simulink model "Hybrid_P2_Parallel"  (R2017b)
settings: Solver=FixedStepAuto  StartTime=0.0  StopTime=length(Speed)  FixedStep=0.01  MaxStep=0.01  RelTol=1e-3  EnableMultiTasking=on
PostLoadFcn:
  | , if any(exist('dsrtsu_mdlpostloadfcn', 'file') == [2, 3, 6]), try dsrtsu_mdlpostloadfcn('Execute', bdroot); catch fprintf('Error in PostLoadFcn (dsrtsu_mdlpostloadfcn) for model "%s":\n %s\n', bdroot, lasterr); end, end,
undefined symbols (not defined in the file): APP1_OOR, APP2_OOR, APP_Mismatch, Brk_Flt, cal, clt, Clutch, Clutch2, ClutchEngag, eng, Engine, EngOverTemp, ENGTRQ_MSMCH_Degraded_CP, ENGTRQ_MSMCH_ErrCritical_CP, ENGTRQ_MSMCH_LimpHome_CP, EngTrqMismatch, ess, ESSOverTemp, gb, KeyPos_Flt, LossCAN, MCUOverTemp, mot, MotDirMismatch, MotOverTemp, MotTrqMismatch, mph2kph, PRNDL_Flt, RegenFault, time, tloop
libraries: simulink x100, EC2_libraries x7, powerlib_meascontrol x2, lib_Actuators x1, CalculationGallon x1, lib_Chassis x1, autolibcoupling x1, autolibsharedcoupling x1, lib_DCDC x1, lib_Differential x1, lib_EMachine_2017a x1, lib_HVESS x1
(part 4 of 7)

== system Hybrid_P2_Parallel/Controller/HSC/Powertrain Manager/Torque Distribution/Supervisory  Control  Logic/VehReady.CS_Mode.Engine_Charge.Brake_mode1.MotTrqCalc1 ==
  note: Regenerative braking:
      | Regenerative braking should be allowed under specific chassis speed:
      | chas_spd_below_no_regen= 1.5;
      | chas_spd_above_full_regen = 3;
      | ess_soc_above_regen_forbidden = .92;  % ESS SOC above which regen braking is forbidden
      | ess_soc_above_regen_allowed = .9;% ESS SOC above which regen braking is allowed
  BPP : Inport
  VehSpd : Inport  Port=2
  ShftLvrPos : Inport  Port=3
  MotSpeed : Inport  Port=4
  TransRatio : Inport  Port=5
  IntdAxleTrq : Inport  Port=6
  f : TriggerPort  TriggerType=function-call  VariantControl=Variant
      settings: CopyFcn=Stateflow.SLINSF.SimulinkMan.removeBlockPreDeleteFcn  PreDeleteFcn=Stateflow.SLINSF.SimulinkMan.unsafePredeleteFcn
  "% to 1 " : Gain  Gain=1/100
  Constant : Constant  Value=0
  Constant1 : Constant  Value=0
  Constant2 : Constant  Value=fd.plant.init.ratio
  Divide : Product  Inputs=***
  Divide2 : Product  Inputs=***
  Index Vector : MultiPortSwitch  DataPortOrder=Zero-based contiguous  Inputs=5  zeroidx=on
  MinMax : MinMax  Function=max  Inputs=2
  Peak trq max - Regen : Lookup  InputValues=mot.plant.init.regen.trq_max.idx1_spd  Table=mot.plant.init.regen.trq_max.map  LookUpMeth=Interpolation-Use End Values  SaturateOnIntegerOverflow=on
  Regen Trq Derating1 : Lookup_n-D  NumberOfTableDimensions=1  BreakpointsForDimension1=[0 10 11 200]  Table=[0 0.5 1 1]  ExtrapMethod=Clip  UseLastTableValue=on  InternalRulePriority=Speed  RndMeth=Simplest  InputSameDT=on
  Regen_derat_overri : Constant  Value=0
  Regen_derat_value : Constant  Value=0.5
  Switch : Switch  Criteria=u2 > Threshold
  limit to 100Nm : Saturate  UpperLimit=0  LowerLimit=-100
  T : Outport
  wires:
  MinMax/1 -> [TrqCalc]
  IntdAxleTrq/1 -> MinMax/1
  Regen_derat_value/1 -> Switch/1
  Switch/1 -> Divide/3
  Regen_derat_overri/1 -> Switch/2
  Regen Trq Derating1/1 -> Switch/3
  Divide2/1 -> MinMax/2  "motor"
  TransRatio/1 -> Divide2/3
  limit to 100Nm/1 -> Divide2/2
  Constant2/1 -> Divide2/1
  Peak trq max - Regen/1 -> Divide/2
  MotSpeed/1 -> Peak trq max - Regen/1  "RPM"
  [TrqCalc] -> Index Vector/5  "N"
  Constant1/1 -> Index Vector/3  "P"
  Constant/1 -> Index Vector/2  "Between Ranges"
  Index Vector/1 -> T/1
  [TrqCalc] -> Index Vector/6  "D"
  [TrqCalc] -> Index Vector/4  "R"
  ShftLvrPos/1 -> Index Vector/1
  VehSpd/1 -> Regen Trq Derating1/1
  Divide/1 -> limit to 100Nm/1
  "% to 1 "/1 -> Divide/1
  BPP/1 -> "% to 1 "/1

== system Hybrid_P2_Parallel/Controller/HSC/Powertrain Manager/Torque Distribution/Supervisory  Control  Logic/VehReady.CS_Mode.Engine_Charge.Brake_mode1.MotTrqCalc2 ==
  note: Regenerative braking:
      | Regenerative braking should be allowed under specific chassis speed:
      | chas_spd_below_no_regen= 1.5;
      | chas_spd_above_full_regen = 3;
      | ess_soc_above_regen_forbidden = .92;  % ESS SOC above which regen braking is forbidden
      | ess_soc_above_regen_allowed = .9;% ESS SOC above which regen braking is allowed
  ShftLvrPos : Inport
  TransRatio : Inport  Port=2
  f : TriggerPort  TriggerType=function-call  VariantControl=Variant
      settings: CopyFcn=Stateflow.SLINSF.SimulinkMan.removeBlockPreDeleteFcn  PreDeleteFcn=Stateflow.SLINSF.SimulinkMan.unsafePredeleteFcn
  Constant : Constant  Value=0
  Constant1 : Constant  Value=0
  Constant2 : Constant  Value=fd.plant.init.ratio
  Divide2 : Product  Inputs=***
  Idle_torque_Regen : Constant  Value=0
  Index Vector : MultiPortSwitch  DataPortOrder=Zero-based contiguous  Inputs=5  zeroidx=on
  T : Outport
  wires:
  Idle_torque_Regen/1 -> Divide2/2
  Divide2/1 -> [TrqCalc]  "motor"
  TransRatio/1 -> Divide2/3
  Constant2/1 -> Divide2/1
  [TrqCalc] -> Index Vector/5  "N"
  Constant1/1 -> Index Vector/3  "P"
  Constant/1 -> Index Vector/2  "Between Ranges"
  Index Vector/1 -> T/1
  [TrqCalc] -> Index Vector/6  "D"
  [TrqCalc] -> Index Vector/4  "R"
  ShftLvrPos/1 -> Index Vector/1

== system Hybrid_P2_Parallel/Controller/HSC/Powertrain Manager/Torque Distribution/Supervisory  Control  Logic/VehReady.CS_Mode.Engine_Charge.Drive_Mode.EngTrq2EngApp ==
  Trq : Inport
  TransRatio : Inport  Port=2
  f : TriggerPort  TriggerType=function-call  VariantControl=Variant
      settings: CopyFcn=Stateflow.SLINSF.SimulinkMan.removeBlockPreDeleteFcn  PreDeleteFcn=Stateflow.SLINSF.SimulinkMan.unsafePredeleteFcn
  0-100% : Saturate  UpperLimit=100  LowerLimit=0
  Compare To Constant : simulink/Logic and Bit Operations/Compare To Constant  relop===  const=0  OutDataTypeStr=boolean
  Constant1 : Constant  Value=eps
  Constant5 : Constant  Value=fd.plant.init.ratio
  Divide1 : Product  Inputs=*//
  EngTrq2EngAPP : Lookup_n-D  NumberOfTableDimensions=1  BreakpointsForDimension1=[0:1:230]  Table="[-0.950562242591810\t-0.861179388327002\t-0.757792747831397\t-0.640901927898975\t-0.511000095283862\t-0.368573976700328\t-0.214103858822793\t-0.0480635882858183\t0.129079428315885\t0.316864224427463\t0.514836273533913\t0.722547489160089\t0.939556224870697\t1.16542727427030\t1.39973187100331\t1.64204768875400\t1.89195884124648\t2.14905588224475\t2.41293580555262\t2.68320204501379\t2.95946447451180\t3.24133940797003\t3.52844959935174\t3.82042424266002\t4.11689897193784\t4.41751586126800\t4.72192342477317\t5.02977661661586\t5.34073683099846\t5.65447190216317\t5.97065610439209\t6.28897015200715\t6.60910119937013\t6.93074284088268\t7.25359511098630\t7.57736448416234\t7.90176387493200\t8.22651263785634\t8.55133656753627\t8.87596789861257\t9.20014530576584\t9.52361390371657\t9.84612524722509\t10.1674373310916\t10.4873145901561\t10.8055278992985\t11.1218545734385\t11.4360783675358\t11.7479894765898\t12.0573845356398\t12.3640666197649\t12.6678452440843\t12.9685363637566\t13.2659623739808\t13.5599521099953\t13.8503408470787\t14.1369703005491\t14.4196886257647\t14.6983504181235\t14.9728167130634\t15.2429549860620\t15.5086391526369\t15.7697495683456\t16.0261730287853\t16.2778027695931\t16.5245384664460\t16.7662862350608\t17.0029586311942\t17.2344746506427\t17.4607597292427\t17.6817457428705\t17.8973710074422\t18.1075802789137\t18.3123247532808\t18.5115620665792\t18.7052562948843\t18.8933779543117\t19.0759040010164\t19.2528178311935\t19.4241092810781\t19.5897746269448\t19.7498165851084\t19.9042443119232\t20.0530734037837\t20.1963258971241\t20.3340302684184\t20.4662214341804\t20.5929407509641\t20.7142360153630\t20.8301614640105\t20.9407777735800\t21.0461520607847\t21.1463578823776\t21.2414752351516\t21.3315905559394\t21.4167967216136\t21.4971930490867\t21.5728852953111\t21.6439856572787\t21.7106127720217\t21.7728917166119\t21.8309540081611\t21.8849376038208\t21.9349869007824\t21.9812527362772\t22.0238923875764\t22.0630695719909\t22.0989544468717\t22.1317236096093\t22.1615600976344\t22.1886533884173\t22.2131993994684\t22.2354004883376\t22.2554654526151\t22.2736095299306\t22.2900543979538\t22.3050281743942\t22.3187654170013\t22.3315071235641\t22.3435007319120\t22.3550001199137\t22.3662656054781\t22.3775639465539\t22.3891683411296\t22.4013584272335\t22.4144202829338\t22.4286464263386\t22.4443358155959\t22.4617938488934\t22.4813323644587\t22.5032696405595\t22.5279303955028\t22.5556457876361\t22.5867534153463\t22.6215973170604\t22.6605279712450\t22.7039022964069\t22.7520836510924\t22.8054418338880\t22.8643530834197\t22.9292000783536\t23.0003719373956\t23.0782642192915\t23.1632789228268\t23.2558244868269\t23.3563157901571\t23.4651741517227\t23.5828273304686\t23.7097095253797\t23.8462613754808\t23.9929299598362\t24.1501687975506\t24.3184378477682\t24.4982035096730\t24.6899386224892\t24.8941224654804\t25.1112407579505\t25.3417856592430\t25.5862557687413\t25.8451561258686\t26.1189982100880\t26.4082999409026\t26.7135856778550\t27.0353862205281\t27.3742388085443\t27.7306871215661\t28.1052812792955\t28.4985778414748\t28.9111398078859\t29.3435366183506\t29.7963441527305\t30.2701447309271\t30.7655271128819\t31.2830864985759\t31.8234245280303\t32.3871492813060\t32.9748752785038\t33.5872234797643\t34.2248212852680\t34.8883025352352\t35.5783075099261\t36.2954829296408\t37.0404819547192\t37.8139641855409\t38.6165956625258\t39.4490488661331\t40.3120027168621\t41.2061425752523\t42.1321602418824\t43.0907539573713\t44.0826284023780\t45.1084946976008\t46.1690704037782\t47.2650795216887\t48.3972524921501\t49.5663261960208\t50.7730439541983\t52.0181555276205\t53.3024171172650\t54.6265913641491\t55.9914473493301\t57.3977605939052\t58.8463130590113\t60.3378931458253\t61.8732956955639\t63.4533219894835\t65.0787797488808\t66.7504831350916\t68.4692527494924\t70.2359156334991\t72.0513052685674\t73.9162615761929\t75.8316309179113\t77.7982660952979\t79.8170263499681\t81.8887773635766\t84.0143912578187\t86.1947465944290\t88.4307283751822\t90.7232280418928\t93.0731434764153\t95.4813790006436\t97.9488453765121\t100\t100\t100\t100\t100\t100\t100\t100]"  ExtrapMethod=Clip  UseLastTableValue=on  InternalRulePriority=Speed  RndMeth=Simplest  InputSameDT=on
  EngTrq2EngAPP_Linear : Lookup_n-D  NumberOfTableDimensions=1  BreakpointsForDimension1=[0:1:250]  Table=[0:0.4:100]  ExtrapMethod=Clip  UseLastTableValue=on  InternalRulePriority=Speed  RndMeth=Simplest  InputSameDT=on
  Switch : Switch  Criteria=u2 > Threshold
  APP : Outport
  wires:
  EngTrq2EngAPP_Linear/1 -> 0-100%/1  "EngTrq2EngAPP_CS"
  0-100%/1 -> APP/1
  TransRatio/1 -> Compare To Constant/1, Switch/3
  Divide1/1 -> EngTrq2EngAPP_Linear/1
  Switch/1 -> Divide1/3
  Constant1/1 -> Switch/1
  Compare To Constant/1 -> Switch/2
  Constant5/1 -> Divide1/2
  Trq/1 -> Divide1/1  "EngAxlTrqReq_CS"

== system Hybrid_P2_Parallel/Controller/HSC/Powertrain Manager/Torque Distribution/Supervisory  Control  Logic/VehReady.CS_Mode.Engine_Charge.Drive_Mode.EngTrqCalc ==
  EngSpeed : Inport
  APP : Inport  Port=2
  VehSpd : Inport  Port=3
  ShftLvrPos : Inport  Port=4
  DrvIntdAxleTrq : Inport  Port=5
  TransRatio : Inport  Port=6
  SOC : Inport  Port=7
  f : TriggerPort  TriggerType=function-call  VariantControl=Variant
      settings: CopyFcn=Stateflow.SLINSF.SimulinkMan.removeBlockPreDeleteFcn  PreDeleteFcn=Stateflow.SLINSF.SimulinkMan.unsafePredeleteFcn
  APP Derating : Lookup_n-D  NumberOfTableDimensions=1  BreakpointsForDimension1=[0 1 2 3 5 7]  Table=[0 0.1 0.3 0.5 0.7 1]  ExtrapMethod=Clip  UseLastTableValue=on  InternalRulePriority=Speed  RndMeth=Simplest  InputSameDT=on
  Constant : Constant  Value=0
  Constant1 : Constant  Value=0
  Constant3 : Constant  Value=fd.plant.init.ratio
  Divide : Product  Inputs=***
  Divide2 : Product  Inputs=***
  EngOptmTrq_Original : Lookup_n-D  NumberOfTableDimensions=1  BreakpointsForDimension1=[1550 1650 1850 2050 2350 2650 2950 3150 3250 3350]  Table="[154.020912669576\t173.623574282068\t180.662367834043\t186.327738253926\t182.858870786433\t180.175407273844\t178.037732950256\t181.891363533595\t190.985931710274\t199.537540592824]"  ExtrapMethod=Clip  UseLastTableValue=on  InternalRulePriority=Speed  RndMeth=Simplest  InputSameDT=on
  Engine Max Trq : Lookup_n-D  NumberOfTableDimensions=1  BreakpointsForDimension1="[600\t800\t1000\t1200\t1400\t1600\t1800\t2000\t2200\t2400\t2600\t2800\t3000\t3200\t3400\t3600\t3800\t4000\t4250\t4500\t4750\t5000\t5250\t5500\t5750\t6000\t6250\t6500]"  Table="[83.7900000000000\t136.760000000000\t140\t152.010000000000\t171.590000000000\t185.900000000000\t198.400000000000\t197.360000000000\t200.550000000000\t202.260000000000\t215.080000000000\t204.810000000000\t204.520000000000\t208.100000000000\t211.520000000000\t210.560000000000\t214.100000000000\t213.470000000000\t208.730000000000\t208.430000000000\t208.670000000000\t231.210000000000\t228.310000000000\t225.330000000000\t220.520000000000\t211.210000000000\t204.190000000000\t151.770000000000]"  ExtrapMethod=Clip  UseLastTableValue=on  InternalRulePriority=Speed  RndMeth=Simplest  InputSameDT=on
  MinMax : MinMax  Function=max  Inputs=2
  SOC Window Estimation : Subsystem
  Shifter : MultiPortSwitch  DataPortOrder=Zero-based contiguous  Inputs=5  zeroidx=on
  Switch : Switch  Criteria=u2 > Threshold
  VehSpd Derating : Lookup_n-D  NumberOfTableDimensions=1  BreakpointsForDimension1=[0 2 5]  Table=[0 0.5 1]  ExtrapMethod=Clip  UseLastTableValue=on  InternalRulePriority=Speed  RndMeth=Simplest  InputSameDT=on
  Trq : Outport
  EngActTRq : Outport  Port=2
  wires:
  MinMax/1 -> [TrqCalc]  "EngAxlTrqReq_CS"
  Constant3/1 -> Divide2/3
  TransRatio/1 -> Divide2/1
  EngOptmTrq_Original/1 -> Switch/3
  Engine Max Trq/1 -> Switch/1
  SOC Window Estimation/1(Out1) -> Switch/2
  SOC/1 -> SOC Window Estimation/1(SOC)
  Switch/1 -> Divide/1  "EngTrqAvl_CS"
  DrvIntdAxleTrq/1 -> MinMax/1  "DrvIntdAxlTrq_CS"
  Divide2/1 -> MinMax/2, EngActTRq/1  "EngAxlTrqAvl_CS"
  Divide/1 -> Divide2/2
  Shifter/1 -> Trq/1
  [TrqCalc] -> Shifter/5  "N"
  Constant1/1 -> Shifter/3  "P"
  Constant/1 -> Shifter/2  "Between Ranges"
  [TrqCalc] -> Shifter/6  "D"
  [TrqCalc] -> Shifter/4  "R"
  ShftLvrPos/1 -> Shifter/1
  VehSpd Derating/1 -> Divide/3  "VehSpeedDerating_CS"
  VehSpd/1 -> VehSpd Derating/1
  APP Derating/1 -> Divide/2  "APPDerating_CS"
  APP/1 -> APP Derating/1
  EngSpeed/1 -> Engine Max Trq/1, EngOptmTrq_Original/1

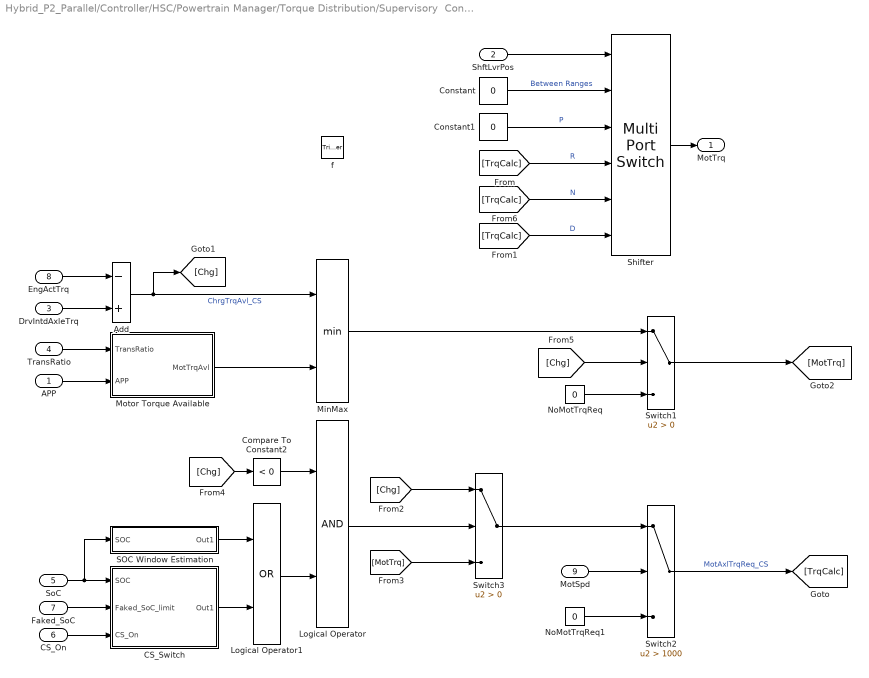
== system Hybrid_P2_Parallel/Controller/HSC/Powertrain Manager/Torque Distribution/Supervisory  Control  Logic/VehReady.CS_Mode.Engine_Charge.Drive_Mode.MotTrqCalc ==
  APP : Inport
  ShftLvrPos : Inport  Port=2
  DrvIntdAxleTrq : Inport  Port=3
  TransRatio : Inport  Port=4
  SoC : Inport  Port=5
  CS_On : Inport  Port=6
  Faked_SoC : Inport  Port=7
  EngActTrq : Inport  Port=8
  MotSpd : Inport  Port=9
  f : TriggerPort  TriggerType=function-call  VariantControl=Variant
      settings: CopyFcn=Stateflow.SLINSF.SimulinkMan.removeBlockPreDeleteFcn  PreDeleteFcn=Stateflow.SLINSF.SimulinkMan.unsafePredeleteFcn
  Add : Sum  Inputs=-+
  CS_Switch : Subsystem
  Compare To Constant2 : simulink/Logic and Bit Operations/Compare To Constant  relop=<  const=0  OutDataTypeStr=boolean
  Constant : Constant  Value=0
  Constant1 : Constant  Value=0
  Logical Operator : Logic  AllPortsSameDT=off  OutDataTypeStr=boolean
  Logical Operator1 : Logic  Operator=OR  AllPortsSameDT=off  OutDataTypeStr=boolean
  MinMax : MinMax  Inputs=2
  Motor Torque Available : Subsystem
  NoMotTrqReq : Constant  Value=0
  NoMotTrqReq1 : Constant  Value=0
  SOC Window Estimation : Subsystem
  Shifter : MultiPortSwitch  DataPortOrder=Zero-based contiguous  Inputs=5  zeroidx=on
  Switch1 : Switch  Criteria=u2 > Threshold
  Switch2 : Switch  Criteria=u2 > Threshold  Threshold=1000
  Switch3 : Switch  Criteria=u2 > Threshold
  MotTrq : Outport
  wires:
  [Chg] -> Switch1/2
  MotSpd/1 -> Switch2/2
  Motor Torque Available/1(MotTrqAvl) -> MinMax/2
  APP/1 -> Motor Torque Available/2(APP)
  TransRatio/1 -> Motor Torque Available/1(TransRatio)
  [Chg] -> Compare To Constant2/1
  [MotTrq] -> Switch3/3
  Switch1/1 -> [MotTrq]
  EngActTrq/1 -> Add/1
  Switch2/1 -> [TrqCalc]  "MotAxlTrqReq_CS"
  NoMotTrqReq1/1 -> Switch2/3
  CS_Switch/1(Out1) -> Logical Operator1/2
  CS_On/1 -> CS_Switch/3(CS_On)
  Faked_SoC/1 -> CS_Switch/2(Faked_SoC_limit)
  SOC Window Estimation/1(Out1) -> Logical Operator1/1
  Logical Operator1/1 -> Logical Operator/2
  Switch3/1 -> Switch2/1
  [Chg] -> Switch3/1
  Logical Operator/1 -> Switch3/2
  Compare To Constant2/1 -> Logical Operator/1
  NoMotTrqReq/1 -> Switch1/3
  MinMax/1 -> Switch1/1
  Add/1 -> MinMax/1, [Chg]  "ChrgTrqAvl_CS"
  SoC/1 -> CS_Switch/1(SOC), SOC Window Estimation/1(SOC)
  DrvIntdAxleTrq/1 -> Add/2
  Shifter/1 -> MotTrq/1
  [TrqCalc] -> Shifter/5  "N"
  Constant1/1 -> Shifter/3  "P"
  Constant/1 -> Shifter/2  "Between Ranges"
  [TrqCalc] -> Shifter/6  "D"
  [TrqCalc] -> Shifter/4  "R"
  ShftLvrPos/1 -> Shifter/1

== system Hybrid_P2_Parallel/Controller/HSC/Powertrain Manager/Torque Distribution/Supervisory  Control  Logic/VehReady.Clutch_Engage.SyncCtrl ==
  EngSpeed : Inport
  MotorSpeed : Inport  Port=2
  f : TriggerPort  TriggerType=function-call  VariantControl=Variant
      settings: CopyFcn=Stateflow.SLINSF.SimulinkMan.removeBlockPreDeleteFcn  PreDeleteFcn=Stateflow.SLINSF.SimulinkMan.unsafePredeleteFcn
  Kp : Gain  Gain=1/50
  Saturation1 : Saturate  UpperLimit=500  LowerLimit=-500
  Sum : Sum  Inputs=|+-
  EngApp : Outport
  wires:
  MotorSpeed/1 -> Sum/1  "RPM"
  EngSpeed/1 -> Sum/2
  Sum/1 -> Kp/1
  Kp/1 -> Saturation1/1
  Saturation1/1 -> EngApp/1

== system Hybrid_P2_Parallel/Controller/HSC/Powertrain Manager/Torque Distribution/Supervisory  Control  Logic/VehReady.Clutch_Engage1.SyncCtrl ==
  EngSpeed : Inport
  MotorSpeed : Inport  Port=2
  f : TriggerPort  TriggerType=function-call  VariantControl=Variant
      settings: CopyFcn=Stateflow.SLINSF.SimulinkMan.removeBlockPreDeleteFcn  PreDeleteFcn=Stateflow.SLINSF.SimulinkMan.unsafePredeleteFcn
  Kp : Gain  Gain=1/100
  Saturation : Saturate  UpperLimit=20  LowerLimit=0
  Sum : Sum  Inputs=|+-
  EngApp : Outport
  wires:
  MotorSpeed/1 -> Sum/1  "RPM"
  EngSpeed/1 -> Sum/2
  Sum/1 -> Kp/1
  Kp/1 -> Saturation/1
  Saturation/1 -> EngApp/1

== system Hybrid_P2_Parallel/Controller/HSC/Powertrain Manager/Torque Distribution/Supervisory  Control  Logic/VehReady.Clutch_Engage2.SyncCtrl ==
  EngSpeed : Inport
  MotorSpeed : Inport  Port=2
  f : TriggerPort  TriggerType=function-call  VariantControl=Variant
      settings: CopyFcn=Stateflow.SLINSF.SimulinkMan.removeBlockPreDeleteFcn  PreDeleteFcn=Stateflow.SLINSF.SimulinkMan.unsafePredeleteFcn
  Kp : Gain  Gain=1/100
  Saturation : Saturate  UpperLimit=20  LowerLimit=0
  Sum : Sum  Inputs=|+-
  EngApp : Outport
  wires:
  MotorSpeed/1 -> Sum/1  "RPM"
  EngSpeed/1 -> Sum/2
  Sum/1 -> Kp/1
  Kp/1 -> Saturation/1
  Saturation/1 -> EngApp/1

== system Hybrid_P2_Parallel/Controller/HSC/Powertrain Manager/Torque Distribution/Supervisory  Control  Logic/VehReady.Clutch_Engage3.SyncCtrl ==
  EngSpeed : Inport
  MotorSpeed : Inport  Port=2
  f : TriggerPort  TriggerType=function-call  VariantControl=Variant
      settings: CopyFcn=Stateflow.SLINSF.SimulinkMan.removeBlockPreDeleteFcn  PreDeleteFcn=Stateflow.SLINSF.SimulinkMan.unsafePredeleteFcn
  Kp : Gain  Gain=1/100
  Saturation : Saturate  UpperLimit=20  LowerLimit=0
  Sum : Sum  Inputs=|+-
  EngApp : Outport
  wires:
  MotorSpeed/1 -> Sum/1  "RPM"
  EngSpeed/1 -> Sum/2
  Sum/1 -> Kp/1
  Kp/1 -> Saturation/1
  Saturation/1 -> EngApp/1

== system Hybrid_P2_Parallel/Controller/HSC/Powertrain Manager/Torque Distribution/Supervisory  Control  Logic/VehReady.Eng_Charging_Stat.EngTrq2EngApp ==
  Trq : Inport
  TransRatio : Inport  Port=2
  f : TriggerPort  TriggerType=function-call  VariantControl=Variant
      settings: CopyFcn=Stateflow.SLINSF.SimulinkMan.removeBlockPreDeleteFcn  PreDeleteFcn=Stateflow.SLINSF.SimulinkMan.unsafePredeleteFcn
  Compare To Constant : simulink/Logic and Bit Operations/Compare To Constant  relop===  const=0  OutDataTypeStr=boolean
  Constant1 : Constant  Value=eps
  Constant5 : Constant  Value=fd.plant.init.ratio
  Divide1 : Product  Inputs=*//
  EngTrq2EngAPP : Lookup_n-D  NumberOfTableDimensions=1  BreakpointsForDimension1=[0:1:230]  Table="[-0.950562242591810\t-0.861179388327002\t-0.757792747831397\t-0.640901927898975\t-0.511000095283862\t-0.368573976700328\t-0.214103858822793\t-0.0480635882858183\t0.129079428315885\t0.316864224427463\t0.514836273533913\t0.722547489160089\t0.939556224870697\t1.16542727427030\t1.39973187100331\t1.64204768875400\t1.89195884124648\t2.14905588224475\t2.41293580555262\t2.68320204501379\t2.95946447451180\t3.24133940797003\t3.52844959935174\t3.82042424266002\t4.11689897193784\t4.41751586126800\t4.72192342477317\t5.02977661661586\t5.34073683099846\t5.65447190216317\t5.97065610439209\t6.28897015200715\t6.60910119937013\t6.93074284088268\t7.25359511098630\t7.57736448416234\t7.90176387493200\t8.22651263785634\t8.55133656753627\t8.87596789861257\t9.20014530576584\t9.52361390371657\t9.84612524722509\t10.1674373310916\t10.4873145901561\t10.8055278992985\t11.1218545734385\t11.4360783675358\t11.7479894765898\t12.0573845356398\t12.3640666197649\t12.6678452440843\t12.9685363637566\t13.2659623739808\t13.5599521099953\t13.8503408470787\t14.1369703005491\t14.4196886257647\t14.6983504181235\t14.9728167130634\t15.2429549860620\t15.5086391526369\t15.7697495683456\t16.0261730287853\t16.2778027695931\t16.5245384664460\t16.7662862350608\t17.0029586311942\t17.2344746506427\t17.4607597292427\t17.6817457428705\t17.8973710074422\t18.1075802789137\t18.3123247532808\t18.5115620665792\t18.7052562948843\t18.8933779543117\t19.0759040010164\t19.2528178311935\t19.4241092810781\t19.5897746269448\t19.7498165851084\t19.9042443119232\t20.0530734037837\t20.1963258971241\t20.3340302684184\t20.4662214341804\t20.5929407509641\t20.7142360153630\t20.8301614640105\t20.9407777735800\t21.0461520607847\t21.1463578823776\t21.2414752351516\t21.3315905559394\t21.4167967216136\t21.4971930490867\t21.5728852953111\t21.6439856572787\t21.7106127720217\t21.7728917166119\t21.8309540081611\t21.8849376038208\t21.9349869007824\t21.9812527362772\t22.0238923875764\t22.0630695719909\t22.0989544468717\t22.1317236096093\t22.1615600976344\t22.1886533884173\t22.2131993994684\t22.2354004883376\t22.2554654526151\t22.2736095299306\t22.2900543979538\t22.3050281743942\t22.3187654170013\t22.3315071235641\t22.3435007319120\t22.3550001199137\t22.3662656054781\t22.3775639465539\t22.3891683411296\t22.4013584272335\t22.4144202829338\t22.4286464263386\t22.4443358155959\t22.4617938488934\t22.4813323644587\t22.5032696405595\t22.5279303955028\t22.5556457876361\t22.5867534153463\t22.6215973170604\t22.6605279712450\t22.7039022964069\t22.7520836510924\t22.8054418338880\t22.8643530834197\t22.9292000783536\t23.0003719373956\t23.0782642192915\t23.1632789228268\t23.2558244868269\t23.3563157901571\t23.4651741517227\t23.5828273304686\t23.7097095253797\t23.8462613754808\t23.9929299598362\t24.1501687975506\t24.3184378477682\t24.4982035096730\t24.6899386224892\t24.8941224654804\t25.1112407579505\t25.3417856592430\t25.5862557687413\t25.8451561258686\t26.1189982100880\t26.4082999409026\t26.7135856778550\t27.0353862205281\t27.3742388085443\t27.7306871215661\t28.1052812792955\t28.4985778414748\t28.9111398078859\t29.3435366183506\t29.7963441527305\t30.2701447309271\t30.7655271128819\t31.2830864985759\t31.8234245280303\t32.3871492813060\t32.9748752785038\t33.5872234797643\t34.2248212852680\t34.8883025352352\t35.5783075099261\t36.2954829296408\t37.0404819547192\t37.8139641855409\t38.6165956625258\t39.4490488661331\t40.3120027168621\t41.2061425752523\t42.1321602418824\t43.0907539573713\t44.0826284023780\t45.1084946976008\t46.1690704037782\t47.2650795216887\t48.3972524921501\t49.5663261960208\t50.7730439541983\t52.0181555276205\t53.3024171172650\t54.6265913641491\t55.9914473493301\t57.3977605939052\t58.8463130590113\t60.3378931458253\t61.8732956955639\t63.4533219894835\t65.0787797488808\t66.7504831350916\t68.4692527494924\t70.2359156334991\t72.0513052685674\t73.9162615761929\t75.8316309179113\t77.7982660952979\t79.8170263499681\t81.8887773635766\t84.0143912578187\t86.1947465944290\t88.4307283751822\t90.7232280418928\t93.0731434764153\t95.4813790006436\t97.9488453765121\t100\t100\t100\t100\t100\t100\t100\t100]"  ExtrapMethod=Clip  UseLastTableValue=on  InternalRulePriority=Speed  RndMeth=Simplest  InputSameDT=on
  Saturation : Saturate  UpperLimit=100  LowerLimit=0
  Switch : Switch  Criteria=u2 > Threshold
  APP : Outport
  wires:
  Saturation/1 -> APP/1
  EngTrq2EngAPP/1 -> Saturation/1
  TransRatio/1 -> Compare To Constant/1, Switch/3
  Divide1/1 -> EngTrq2EngAPP/1
  Switch/1 -> Divide1/3
  Constant1/1 -> Switch/1
  Compare To Constant/1 -> Switch/2
  Constant5/1 -> Divide1/2
  Trq/1 -> Divide1/1

== system Hybrid_P2_Parallel/Controller/HSC/Powertrain Manager/Torque Distribution/Supervisory  Control  Logic/VehReady.Eng_Charging_Stat.EngTrqCalc ==
  EngSpeed : Inport
  ShftLvrPos : Inport  Port=2
  DrvIntdAxleTrq : Inport  Port=3
  TransRatio : Inport  Port=4
  f : TriggerPort  TriggerType=function-call  VariantControl=Variant
      settings: CopyFcn=Stateflow.SLINSF.SimulinkMan.removeBlockPreDeleteFcn  PreDeleteFcn=Stateflow.SLINSF.SimulinkMan.unsafePredeleteFcn
  Constant{,1..2,4} (4 alike) : Constant  Value=0
  Constant3 : Constant  Value=fd.plant.init.ratio
  Divide2 : Product  Inputs=***
  Engine Max Trq : Lookup_n-D  NumberOfTableDimensions=1  BreakpointsForDimension1="[600\t800\t1000\t1200\t1400\t1600\t1800\t2000\t2200\t2400\t2600\t2800\t3000\t3200\t3400\t3600\t3800\t4000\t4250\t4500\t4750\t5000\t5250\t5500\t5750\t6000\t6250\t6500]"  Table="[83.7900000000000\t136.760000000000\t140\t152.010000000000\t171.590000000000\t185.900000000000\t198.400000000000\t197.360000000000\t200.550000000000\t202.260000000000\t215.080000000000\t204.810000000000\t204.520000000000\t208.100000000000\t211.520000000000\t210.560000000000\t214.100000000000\t213.470000000000\t208.730000000000\t208.430000000000\t208.670000000000\t231.210000000000\t228.310000000000\t225.330000000000\t220.520000000000\t211.210000000000\t204.190000000000\t151.770000000000]"  ExtrapMethod=Clip  UseLastTableValue=on  InternalRulePriority=Speed  RndMeth=Simplest  InputSameDT=on
  MinMax : MinMax  Function=max  Inputs=2
  Multiply by Zero Fix : Subsystem
  Shifter : MultiPortSwitch  DataPortOrder=Zero-based contiguous  Inputs=5  zeroidx=on
  Trq : Outport
  wires:
  Multiply by Zero Fix/1(Out1) -> Divide2/3
  TransRatio/1 -> Multiply by Zero Fix/1(In1)
  MinMax/1 -> [TrqCalc]
  DrvIntdAxleTrq/1 -> MinMax/1  "driver"
  Divide2/1 -> MinMax/2  "engine"
  Engine Max Trq/1 -> Divide2/2
  Constant3/1 -> Divide2/1
  Shifter/1 -> Trq/1
  Constant2/1 -> Shifter/5  "N"
  [TrqCalc] -> Shifter/3  "P"
  Constant/1 -> Shifter/2  "Between Ranges"
  Constant4/1 -> Shifter/6  "D"
  Constant1/1 -> Shifter/4  "R"
  ShftLvrPos/1 -> Shifter/1
  EngSpeed/1 -> Engine Max Trq/1

== system Hybrid_P2_Parallel/Controller/HSC/Powertrain Manager/Torque Distribution/Supervisory  Control  Logic/VehReady.Eng_Charging_Stat.MotTrqCalc ==
  ShftLvrPos : Inport
  DrvIntdAxleTrq : Inport  Port=2
  Trq : Inport  Port=3
  f : TriggerPort  TriggerType=function-call  VariantControl=Variant
      settings: CopyFcn=Stateflow.SLINSF.SimulinkMan.removeBlockPreDeleteFcn  PreDeleteFcn=Stateflow.SLINSF.SimulinkMan.unsafePredeleteFcn
  Add : Sum  Inputs=-+
  Constant{,1..3} (4 alike) : Constant  Value=0
  Goto : Goto  Commented=on  GotoTag=TrqCalc
  NoMotTrqReq : Constant  Commented=on  Value=0
  Saturation : Saturate  UpperLimit=100  LowerLimit=-inf
  Shifter : MultiPortSwitch  DataPortOrder=Zero-based contiguous  Inputs=5  zeroidx=on
  Switch1 : Switch  Commented=on  Criteria=u2 > Threshold
  MotTrq : Outport
  wires:
  Saturation/1 -> [TrqCalc]
  Add/1 -> Switch1/2, Switch1/1, Saturation/1
  Switch1/1 -> Goto/1
  Trq/1 -> Add/1
  NoMotTrqReq/1 -> Switch1/3
  DrvIntdAxleTrq/1 -> Add/2
  Shifter/1 -> MotTrq/1
  Constant2/1 -> Shifter/5  "N"
  [TrqCalc] -> Shifter/3  "P"
  Constant/1 -> Shifter/2  "Between Ranges"
  Constant3/1 -> Shifter/6  "D"
  Constant1/1 -> Shifter/4  "R"
  ShftLvrPos/1 -> Shifter/1

== system Hybrid_P2_Parallel/Controller/HSC/Powertrain Manager/Torque Distribution/Supervisory  Control  Logic/VehReady.Eng_Only_Mode.EngTrq2EngApp ==
  T : Inport
  TransRatio : Inport  Port=2
  f : TriggerPort  TriggerType=function-call  VariantControl=Variant
      settings: CopyFcn=Stateflow.SLINSF.SimulinkMan.removeBlockPreDeleteFcn  PreDeleteFcn=Stateflow.SLINSF.SimulinkMan.unsafePredeleteFcn
  0-100% : Saturate  UpperLimit=100  LowerLimit=0
  Compare To Constant : simulink/Logic and Bit Operations/Compare To Constant  relop===  const=0  OutDataTypeStr=boolean
  Constant1 : Constant  Value=eps
  Constant5 : Constant  Value=fd.plant.init.ratio
  Divide by 0 Fix : Switch  Criteria=u2 > Threshold
  Divide1 : Product  Inputs=*//
  EngTrq2EngAPP : Lookup_n-D  NumberOfTableDimensions=1  BreakpointsForDimension1=[0:1:230]  Table="[-0.950562242591810\t-0.861179388327002\t-0.757792747831397\t-0.640901927898975\t-0.511000095283862\t-0.368573976700328\t-0.214103858822793\t-0.0480635882858183\t0.129079428315885\t0.316864224427463\t0.514836273533913\t0.722547489160089\t0.939556224870697\t1.16542727427030\t1.39973187100331\t1.64204768875400\t1.89195884124648\t2.14905588224475\t2.41293580555262\t2.68320204501379\t2.95946447451180\t3.24133940797003\t3.52844959935174\t3.82042424266002\t4.11689897193784\t4.41751586126800\t4.72192342477317\t5.02977661661586\t5.34073683099846\t5.65447190216317\t5.97065610439209\t6.28897015200715\t6.60910119937013\t6.93074284088268\t7.25359511098630\t7.57736448416234\t7.90176387493200\t8.22651263785634\t8.55133656753627\t8.87596789861257\t9.20014530576584\t9.52361390371657\t9.84612524722509\t10.1674373310916\t10.4873145901561\t10.8055278992985\t11.1218545734385\t11.4360783675358\t11.7479894765898\t12.0573845356398\t12.3640666197649\t12.6678452440843\t12.9685363637566\t13.2659623739808\t13.5599521099953\t13.8503408470787\t14.1369703005491\t14.4196886257647\t14.6983504181235\t14.9728167130634\t15.2429549860620\t15.5086391526369\t15.7697495683456\t16.0261730287853\t16.2778027695931\t16.5245384664460\t16.7662862350608\t17.0029586311942\t17.2344746506427\t17.4607597292427\t17.6817457428705\t17.8973710074422\t18.1075802789137\t18.3123247532808\t18.5115620665792\t18.7052562948843\t18.8933779543117\t19.0759040010164\t19.2528178311935\t19.4241092810781\t19.5897746269448\t19.7498165851084\t19.9042443119232\t20.0530734037837\t20.1963258971241\t20.3340302684184\t20.4662214341804\t20.5929407509641\t20.7142360153630\t20.8301614640105\t20.9407777735800\t21.0461520607847\t21.1463578823776\t21.2414752351516\t21.3315905559394\t21.4167967216136\t21.4971930490867\t21.5728852953111\t21.6439856572787\t21.7106127720217\t21.7728917166119\t21.8309540081611\t21.8849376038208\t21.9349869007824\t21.9812527362772\t22.0238923875764\t22.0630695719909\t22.0989544468717\t22.1317236096093\t22.1615600976344\t22.1886533884173\t22.2131993994684\t22.2354004883376\t22.2554654526151\t22.2736095299306\t22.2900543979538\t22.3050281743942\t22.3187654170013\t22.3315071235641\t22.3435007319120\t22.3550001199137\t22.3662656054781\t22.3775639465539\t22.3891683411296\t22.4013584272335\t22.4144202829338\t22.4286464263386\t22.4443358155959\t22.4617938488934\t22.4813323644587\t22.5032696405595\t22.5279303955028\t22.5556457876361\t22.5867534153463\t22.6215973170604\t22.6605279712450\t22.7039022964069\t22.7520836510924\t22.8054418338880\t22.8643530834197\t22.9292000783536\t23.0003719373956\t23.0782642192915\t23.1632789228268\t23.2558244868269\t23.3563157901571\t23.4651741517227\t23.5828273304686\t23.7097095253797\t23.8462613754808\t23.9929299598362\t24.1501687975506\t24.3184378477682\t24.4982035096730\t24.6899386224892\t24.8941224654804\t25.1112407579505\t25.3417856592430\t25.5862557687413\t25.8451561258686\t26.1189982100880\t26.4082999409026\t26.7135856778550\t27.0353862205281\t27.3742388085443\t27.7306871215661\t28.1052812792955\t28.4985778414748\t28.9111398078859\t29.3435366183506\t29.7963441527305\t30.2701447309271\t30.7655271128819\t31.2830864985759\t31.8234245280303\t32.3871492813060\t32.9748752785038\t33.5872234797643\t34.2248212852680\t34.8883025352352\t35.5783075099261\t36.2954829296408\t37.0404819547192\t37.8139641855409\t38.6165956625258\t39.4490488661331\t40.3120027168621\t41.2061425752523\t42.1321602418824\t43.0907539573713\t44.0826284023780\t45.1084946976008\t46.1690704037782\t47.2650795216887\t48.3972524921501\t49.5663261960208\t50.7730439541983\t52.0181555276205\t53.3024171172650\t54.6265913641491\t55.9914473493301\t57.3977605939052\t58.8463130590113\t60.3378931458253\t61.8732956955639\t63.4533219894835\t65.0787797488808\t66.7504831350916\t68.4692527494924\t70.2359156334991\t72.0513052685674\t73.9162615761929\t75.8316309179113\t77.7982660952979\t79.8170263499681\t81.8887773635766\t84.0143912578187\t86.1947465944290\t88.4307283751822\t90.7232280418928\t93.0731434764153\t95.4813790006436\t97.9488453765121\t100\t100\t100\t100\t100\t100\t100\t100]"  ExtrapMethod=Clip  UseLastTableValue=on  InternalRulePriority=Speed  RndMeth=Simplest  InputSameDT=on
  APP : Outport
  wires:
  0-100%/1 -> APP/1
  EngTrq2EngAPP/1 -> 0-100%/1
  TransRatio/1 -> Compare To Constant/1, Divide by 0 Fix/3
  Divide1/1 -> EngTrq2EngAPP/1
  Divide by 0 Fix/1 -> Divide1/3
  Constant1/1 -> Divide by 0 Fix/1
  Compare To Constant/1 -> Divide by 0 Fix/2
  Constant5/1 -> Divide1/2
  T/1 -> Divide1/1

== system Hybrid_P2_Parallel/Controller/HSC/Powertrain Manager/Torque Distribution/Supervisory  Control  Logic/VehReady.Eng_Only_Mode.EngTrqCalc ==
  APP : Inport
  EngSpeed : Inport  Port=2
  Shifter : Inport  Port=3
  DrvIntdAxleTrq : Inport  Port=4
  TransRatio : Inport  Port=5
  f : TriggerPort  TriggerType=function-call  VariantControl=Variant
      settings: CopyFcn=Stateflow.SLINSF.SimulinkMan.removeBlockPreDeleteFcn  PreDeleteFcn=Stateflow.SLINSF.SimulinkMan.unsafePredeleteFcn
  Constant : Constant  Value=0
  Constant1 : Constant  Value=0
  Constant2 : Constant  Value=0
  Divide2 : Product  Inputs=**
  Divide3 : Product  Inputs=***
  Engine Max Trq : Lookup_n-D  NumberOfTableDimensions=1  BreakpointsForDimension1="[600\t800\t1000\t1200\t1400\t1600\t1800\t2000\t2200\t2400\t2600\t2800\t3000\t3200\t3400\t3600\t3800\t4000\t4250\t4500\t4750\t5000\t5250\t5500\t5750\t6000\t6250\t6500]"  Table="[83.7900000000000\t136.760000000000\t140\t152.010000000000\t171.590000000000\t185.900000000000\t198.400000000000\t197.360000000000\t200.550000000000\t202.260000000000\t215.080000000000\t204.810000000000\t204.520000000000\t208.100000000000\t211.520000000000\t210.560000000000\t214.100000000000\t213.470000000000\t208.730000000000\t208.430000000000\t208.670000000000\t231.210000000000\t228.310000000000\t225.330000000000\t220.520000000000\t211.210000000000\t204.190000000000\t151.770000000000]"  ExtrapMethod=Clip  UseLastTableValue=on  InternalRulePriority=Speed  RndMeth=Simplest  InputSameDT=on
  Final Drive Ratio1 : Constant  Value=fd.plant.init.ratio
  Gain : Gain  Gain=1/100
  Index Vector : MultiPortSwitch  DataPortOrder=Zero-based contiguous  Inputs=5  zeroidx=on
  MinMax : MinMax  Inputs=2
  T : Outport
  wires:
  MinMax/1 -> [TrqCalc]
  DrvIntdAxleTrq/1 -> MinMax/2
  Divide3/1 -> MinMax/1
  Final Drive Ratio1/1 -> Divide3/3
  TransRatio/1 -> Divide3/2
  Divide2/1 -> Divide3/1
  Engine Max Trq/1 -> Divide2/2
  EngSpeed/1 -> Engine Max Trq/1  "RPM"
  Gain/1 -> Divide2/1
  APP/1 -> Gain/1
  Shifter/1 -> Index Vector/1
  Index Vector/1 -> T/1
  Constant2/1 -> Index Vector/5  "N"
  Constant1/1 -> Index Vector/3  "P"
  Constant/1 -> Index Vector/2  "Between Ranges"
  [TrqCalc] -> Index Vector/6  "D"
  [TrqCalc] -> Index Vector/4  "R"

== system Hybrid_P2_Parallel/Controller/HSC/Powertrain Manager/Torque Distribution/Supervisory  Control  Logic/VehReady.Sport_Mode.Brake_mode.MotTrqCalc1 ==
  note: Regenerative braking:
      | Regenerative braking should be allowed under specific chassis speed:
      | chas_spd_below_no_regen= 1.5;
      | chas_spd_above_full_regen = 3;
      | ess_soc_above_regen_forbidden = .92;  % ESS SOC above which regen braking is forbidden
      | ess_soc_above_regen_allowed = .9;% ESS SOC above which regen braking is allowed
  BPP : Inport
  VehSpd : Inport  Port=2
  ShftLvrPos : Inport  Port=3
  MotSpeed : Inport  Port=4
  IntdAxleTrq : Inport  Port=5
  TransRatio : Inport  Port=6
  f : TriggerPort  TriggerType=function-call  VariantControl=Variant
      settings: CopyFcn=Stateflow.SLINSF.SimulinkMan.removeBlockPreDeleteFcn  PreDeleteFcn=Stateflow.SLINSF.SimulinkMan.unsafePredeleteFcn
  "% to 1 " : Gain  Gain=1/100
  Constant : Constant  Value=0
  Constant1 : Constant  Value=0
  Constant2 : Constant  Value=fd.plant.init.ratio
  Divide : Product  Inputs=***
  Divide2 : Product  Inputs=***
  Index Vector : MultiPortSwitch  DataPortOrder=Zero-based contiguous  Inputs=5  zeroidx=on
  MinMax : MinMax  Function=max  Inputs=2
  Peak trq max - Regen : Lookup  InputValues=mot.plant.init.regen.trq_max.idx1_spd  Table=mot.plant.init.regen.trq_max.map  LookUpMeth=Interpolation-Use End Values  SaturateOnIntegerOverflow=on
  Regen Trq Derating : Lookup_n-D  NumberOfTableDimensions=1  BreakpointsForDimension1=[0 10 20 30 40]  Table=[0 0.025 0.05 0.1 1]  ExtrapMethod=Clip  UseLastTableValue=on  InternalRulePriority=Speed  RndMeth=Simplest  InputSameDT=on
  limit to 200Nm : Saturate  UpperLimit=0  LowerLimit=-200
  T : Outport
  wires:
  Regen Trq Derating/1 -> Divide/3
  MinMax/1 -> [TrqCalc]
  Divide2/1 -> MinMax/2  "motor"
  IntdAxleTrq/1 -> MinMax/1
  TransRatio/1 -> Divide2/3
  limit to 200Nm/1 -> Divide2/2
  Constant2/1 -> Divide2/1
  Peak trq max - Regen/1 -> Divide/2
  MotSpeed/1 -> Peak trq max - Regen/1  "RPM"
  [TrqCalc] -> Index Vector/5  "N"
  Constant1/1 -> Index Vector/3  "P"
  Constant/1 -> Index Vector/2  "Between Ranges"
  Index Vector/1 -> T/1
  [TrqCalc] -> Index Vector/6  "D"
  [TrqCalc] -> Index Vector/4  "R"
  ShftLvrPos/1 -> Index Vector/1
  VehSpd/1 -> Regen Trq Derating/1
  Divide/1 -> limit to 200Nm/1
  "% to 1 "/1 -> Divide/1
  BPP/1 -> "% to 1 "/1

== system Hybrid_P2_Parallel/Controller/HSC/Powertrain Manager/Torque Distribution/Supervisory  Control  Logic/VehReady.Sport_Mode.EngTrq2EngApp ==
  note: Change pedal map
  Trq : Inport
  TransRatio : Inport  Port=2
  f : TriggerPort  TriggerType=function-call  VariantControl=Variant
      settings: CopyFcn=Stateflow.SLINSF.SimulinkMan.removeBlockPreDeleteFcn  PreDeleteFcn=Stateflow.SLINSF.SimulinkMan.unsafePredeleteFcn
  0-100% : Saturate  UpperLimit=100  LowerLimit=0
  Compare To Constant : simulink/Logic and Bit Operations/Compare To Constant  relop===  const=0  OutDataTypeStr=boolean
  Constant1 : Constant  Value=eps
  Constant5 : Constant  Value=fd.plant.init.ratio
  Divide by 0 Fix : Switch  Criteria=u2 > Threshold
  Divide1 : Product  Inputs=*//
  EngTrq2EngAPP_Linear : Lookup_n-D  NumberOfTableDimensions=1  BreakpointsForDimension1=[0:1:200]  Table=[0:0.5:100]  ExtrapMethod=Clip  UseLastTableValue=on  InternalRulePriority=Speed  RndMeth=Simplest  InputSameDT=on
  APP : Outport
  wires:
  EngTrq2EngAPP_Linear/1 -> 0-100%/1
  0-100%/1 -> APP/1
  TransRatio/1 -> Compare To Constant/1, Divide by 0 Fix/3
  Divide1/1 -> EngTrq2EngAPP_Linear/1
  Divide by 0 Fix/1 -> Divide1/3
  Constant1/1 -> Divide by 0 Fix/1
  Compare To Constant/1 -> Divide by 0 Fix/2
  Constant5/1 -> Divide1/2
  Trq/1 -> Divide1/1

== system Hybrid_P2_Parallel/Controller/HSC/Powertrain Manager/Torque Distribution/Supervisory  Control  Logic/VehReady.Sport_Mode.EngTrqCalc ==
  APP : Inport
  EngSpeed : Inport  Port=2
  Shifter : Inport  Port=3
  DrvIntdAxleTrq : Inport  Port=4
  TransRatio : Inport  Port=5
  f : TriggerPort  TriggerType=function-call  VariantControl=Variant
      settings: CopyFcn=Stateflow.SLINSF.SimulinkMan.removeBlockPreDeleteFcn  PreDeleteFcn=Stateflow.SLINSF.SimulinkMan.unsafePredeleteFcn
  Constant : Constant  Value=0
  Constant1 : Constant  Value=0
  Divide2 : Product  Inputs=**
  Divide3 : Product  Inputs=***
  Engine Max Trq : Lookup_n-D  NumberOfTableDimensions=1  BreakpointsForDimension1="[600\t800\t1000\t1200\t1400\t1600\t1800\t2000\t2200\t2400\t2600\t2800\t3000\t3200\t3400\t3600\t3800\t4000\t4250\t4500\t4750\t5000\t5250\t5500\t5750\t6000\t6250\t6500]"  Table="[83.7900000000000\t136.760000000000\t140\t152.010000000000\t171.590000000000\t185.900000000000\t198.400000000000\t197.360000000000\t200.550000000000\t202.260000000000\t215.080000000000\t204.810000000000\t204.520000000000\t208.100000000000\t211.520000000000\t210.560000000000\t214.100000000000\t213.470000000000\t208.730000000000\t208.430000000000\t208.670000000000\t231.210000000000\t228.310000000000\t225.330000000000\t220.520000000000\t211.210000000000\t204.190000000000\t151.770000000000]"  ExtrapMethod=Clip  UseLastTableValue=on  InternalRulePriority=Speed  RndMeth=Simplest  InputSameDT=on
  Final Drive Ratio : Constant  Value=fd.plant.init.ratio
  Index Vector : MultiPortSwitch  DataPortOrder=Zero-based contiguous  Inputs=5  zeroidx=on
  MinMax : MinMax  Inputs=2
  Saturation : Saturate  UpperLimit=230  LowerLimit=-inf
  to% : Gain  Gain=1/100
  T : Outport
  wires:
  [TrqCalc] -> Index Vector/4  "R"
  [TrqCalc] -> Index Vector/6  "D"
  Constant/1 -> Index Vector/2  "Between Ranges"
  Constant1/1 -> Index Vector/3  "P"
  [TrqCalc] -> Index Vector/5  "N"
  Index Vector/1 -> T/1
  Shifter/1 -> Index Vector/1
  APP/1 -> to%/1
  to%/1 -> Divide2/1
  EngSpeed/1 -> Engine Max Trq/1  "RPM"
  Engine Max Trq/1 -> Saturation/1
  Saturation/1 -> Divide2/2
  Divide2/1 -> Divide3/1
  TransRatio/1 -> Divide3/2
  Final Drive Ratio/1 -> Divide3/3
  Divide3/1 -> MinMax/1
  DrvIntdAxleTrq/1 -> MinMax/2
  MinMax/1 -> [TrqCalc]

== system Hybrid_P2_Parallel/Controller/HSC/Powertrain Manager/Torque Distribution/Supervisory  Control  Logic/VehReady.Sport_Mode.MotTrqCalc ==
  APP : Inport
  Shifter : Inport  Port=2
  MotSpeed : Inport  Port=3
  DrvIntdAxleTrq : Inport  Port=4
  TransRatio : Inport  Port=5
  f : TriggerPort  TriggerType=function-call  VariantControl=Variant
      settings: CopyFcn=Stateflow.SLINSF.SimulinkMan.removeBlockPreDeleteFcn  PreDeleteFcn=Stateflow.SLINSF.SimulinkMan.unsafePredeleteFcn
  % to 1 : Gain  Gain=1/100
  Constant : Constant  Value=0
  Constant1 : Constant  Value=0
  Differential Ratio : Constant  Value=fd.plant.init.ratio
  Divide1 : Product  Inputs=**
  Divide2 : Product  Inputs=***
  Index Vector : MultiPortSwitch  DataPortOrder=Zero-based contiguous  Inputs=5  zeroidx=on
  MinMax : MinMax  Inputs=2
  Peak trq max - Motoring : Lookup  InputValues=mot.plant.init.regen.trq_max.idx1_spd  Table=mot.plant.init.motor.trq_max.map  LookUpMeth=Interpolation-Use End Values  SaturateOnIntegerOverflow=on
  T : Outport
  wires:
  % to 1/1 -> Divide1/2
  Shifter/1 -> Index Vector/1
  [TrqCalc] -> Index Vector/4  "R"
  [TrqCalc] -> Index Vector/6  "D"
  Index Vector/1 -> T/1
  Constant/1 -> Index Vector/2  "Between Ranges"
  Constant1/1 -> Index Vector/3  "P"
  [TrqCalc] -> Index Vector/5  "N"
  APP/1 -> % to 1/1
  MotSpeed/1 -> Peak trq max - Motoring/1  "RPM"
  Peak trq max - Motoring/1 -> Divide1/1
  Divide1/1 -> Divide2/1
  TransRatio/1 -> Divide2/2
  Differential Ratio/1 -> Divide2/3
  DrvIntdAxleTrq/1 -> MinMax/1
  Divide2/1 -> MinMax/2
  MinMax/1 -> [TrqCalc]

== system Hybrid_P2_Parallel/Controller/HSC/Powertrain Manager/Torque Distribution/SysPwrMd ==
  note: Switch added to test engine start
      | 04/13/2017 - Sebastian
  note: Disable Engine if HVIL on
  SysPwrMd : Inport
  EngRunAtv : Inport  Port=2
  EngOnReq : Inport  Port=3
  Fehler_Pilot : Inport  Port=4
  Constant1 : Constant  Value=3
  Constant2 : Constant
  Constant3 : Constant  Value=0
  EngOnReq_Cal : Constant  Value=0
  Saturation2 : Saturate  UpperLimit=2  LowerLimit=0
  Saturation3 : Saturate  UpperLimit=2  LowerLimit=0
  Switch{1..5} (5 alike) : Switch  Threshold=1
  Out1 : Outport
  wires:
  Constant3/1 -> Switch5/1
  Switch5/1 -> Out1/1
  Fehler_Pilot/1 -> Switch5/2
  Switch4/1 -> Switch3/2
  EngOnReq_Cal/1 -> Switch4/1, Switch4/2
  Switch3/1 -> Switch5/3
  Switch1/1 -> Switch3/1
  EngOnReq/1 -> Switch4/3
  Saturation3/1 -> Switch2/3
  SysPwrMd/1 -> Saturation2/1, Saturation3/1
  Saturation2/1 -> Switch1/1
  EngRunAtv/1 -> Switch1/2, Switch2/2
  Constant2/1 -> Switch2/1
  Constant1/1 -> Switch1/3
  Switch2/1 -> Switch3/3

== system Hybrid_P2_Parallel/Controller/HSC/Powertrain Manager/Torque Distribution/eSystemStatusValidity ==
  In1 : Inport
  " Normal Operation" : simulink/Logic and Bit Operations/Compare To Constant  relop===  const=2  OutDataTypeStr=boolean
  Limited Operation : simulink/Logic and Bit Operations/Compare To Constant  relop===  const=1  OutDataTypeStr=boolean
  Logical Operator : Logic  Operator=OR  AllPortsSameDT=off  OutDataTypeStr=boolean
  Out1 : Outport
  wires:
  Logical Operator/1 -> Out1/1
  " Normal Operation"/1 -> Logical Operator/2
  Limited Operation/1 -> Logical Operator/1
  In1/1 -> Limited Operation/1, " Normal Operation"/1

== system Hybrid_P2_Parallel/Controller/HSC/Powertrain Manager/Torque Distribution/iceSystemStatusValidity ==
  In1 : Inport
  " Normal Operation" : simulink/Logic and Bit Operations/Compare To Constant  relop===  const=2  OutDataTypeStr=boolean
  Limited Operation : simulink/Logic and Bit Operations/Compare To Constant  relop===  const=1  OutDataTypeStr=boolean
  Logical Operator : Logic  Operator=OR  AllPortsSameDT=off  OutDataTypeStr=boolean
  Out1 : Outport
  wires:
  In1/1 -> " Normal Operation"/1, Limited Operation/1
  Limited Operation/1 -> Logical Operator/1
  " Normal Operation"/1 -> Logical Operator/2
  Logical Operator/1 -> Out1/1

== system Hybrid_P2_Parallel/Controller/HSC/Camaro Fault Detection/Component Diagnostic/Engine Component Diagnostic/Override  engTrqCmd ==
  note: Override Switch Subsystem
  note: This subsystem is used to override the model value of a signal to a constant value
  In1 : Inport
  Constant : Constant  Value=50
  Multiport Switch : MultiPortSwitch  DataPortOrder=Zero-based contiguous  Inputs=2  zeroidx=on
  Signal Override Switch 0 = Use Model 1 = Use Constant : Constant
  Out1 : Outport
  wires:
  Constant/1 -> Multiport Switch/3
  Multiport Switch/1 -> Out1/1
  In1/1 -> Multiport Switch/2
  Signal Override Switch 0 = Use Model 1 = Use Constant/1 -> Multiport Switch/1

== system Hybrid_P2_Parallel/Controller/HSC/Camaro Fault Detection/Component Diagnostic/Engine Component Diagnostic/TorqMismatch Detection ==
  In1 : Inport
  In2 : Inport  Port=2
  In3 : Inport  Port=3
  Abs : Abs
  Add : Sum  Inputs=+-
  Bus Creator : BusCreator  Inputs=3
  Constant : Constant  Value=cal.ENGTRQ_MSMCH.ErrCritical_CP
  Constant1 : Constant  Value=50
  Constant2 : Constant  Value=cal.ENGTRQ_MSMCH.Degraded_CP
  Constant3 : Constant  Value=cal.ENGTRQ_MSMCH.LimpHome_CP
  Constant4 : Constant  Value=0
  Constant5 : Constant  Value=0
  Constant6 : Constant  Value=0
  Data Type Conversion : DataTypeConversion  OutDataTypeStr=boolean
  Data Type Conversion1 : DataTypeConversion  OutDataTypeStr=boolean
  Data Type Conversion2 : DataTypeConversion  OutDataTypeStr=boolean
  Relational Operator : RelationalOperator  OutDataTypeStr=boolean  RndMeth=Nearest
  Relational Operator1 : RelationalOperator  Operator=>  OutDataTypeStr=boolean  RndMeth=Nearest
  Relational Operator2 : RelationalOperator  Operator=>  OutDataTypeStr=boolean  RndMeth=Nearest
  Switch : Switch  Threshold=1
  Terminator{,1..3} (4 alike) : Terminator
  Unit Delay : UnitDelay  Commented=through  SampleTime=-1
  Unit Delay1 : UnitDelay  Commented=through  SampleTime=-1
  "Zero " : Constant  Value=0
  Eng_Torque_Mismch : Outport
  wires:
  Data Type Conversion2/1 -> Bus Creator/3  "Eng_Torque_Mismch_Limp"
  Data Type Conversion1/1 -> Bus Creator/2  "Eng_Torque_Mismch_Degrad"
  Data Type Conversion/1 -> Bus Creator/1  "Eng_Torque_Mismch_Critical"
  Constant5/1 -> Data Type Conversion1/1  "Eng_Torque_Mismch_Degrad"
  Constant6/1 -> Data Type Conversion2/1  "Eng_Torque_Mismch_Limp"
  Constant4/1 -> Data Type Conversion/1  "Eng_Torque_Mismch_Critical"
  Abs/1 -> Relational Operator/1
  Unit Delay1/1 -> Add/2
  Bus Creator/1 -> Eng_Torque_Mismch/1
  Relational Operator2/1 -> Terminator2/1  "Eng_Torque_Mismch_Limp"
  Relational Operator1/1 -> Terminator1/1  "Eng_Torque_Mismch_Degrad"
  Constant3/1 -> Relational Operator2/2
  Constant2/1 -> Relational Operator1/2
  Switch/1 -> Terminator/1, Relational Operator1/1, Relational Operator2/1  "Eng_Torque_Mismch_Critical"
  Relational Operator/1 -> Switch/1
  Add/1 -> Abs/1
  Constant/1 -> Relational Operator/2
  Unit Delay/1 -> Add/1
  In3/1 -> Switch/2
  "Zero "/1 -> Switch/3
  In2/1 -> Unit Delay1/1
  In1/1 -> Unit Delay/1
  Constant1/1 -> Terminator3/1

== system Hybrid_P2_Parallel/Controller/HSC/Camaro Fault Detection/Input Conversions/BMS_Conversions/Override  BMS_gdf 0_1 ==
  note: This subsystem is used to override the model value of a signal to a constant value
  note: Override Switch Subsystem
  In1 : Inport
  Multiport Switch : MultiPortSwitch  DataPortOrder=Zero-based contiguous  Inputs=2  zeroidx=on
  Override Value : Constant  Value=0  OutDataTypeStr=double
  Signal Override Switch 0 = Use Model 1 = Use Constant : Constant
  Out1 : Outport
  wires:
  Signal Override Switch 0 = Use Model 1 = Use Constant/1 -> Multiport Switch/1
  In1/1 -> Multiport Switch/2
  Multiport Switch/1 -> Out1/1
  Override Value/1 -> Multiport Switch/3
